simulink model "connecttoUDP_Ask_For_Ball"  (R2025a)
settings: Solver=ode4  StartTime=0.0  StopTime=inf  FixedStep=1/500  RelTol=1e-3  EnableMultiTasking=on
InitFcn:
  | home = [0.45; 0; 0.49];
  | pick = [0.3; 0; 0.3];
  | place = [-0.25; -0.25; 0.01];
  | waypoints = ...
  | [pick, pick,place ,place ,home]' ;
undefined symbols (not defined in the file): HIL, qc_get_step_size
libraries: quarc_library x18, simulink x3
(part 1 of 2)
settings Model: SimulationMode=external  ExtModeTrigDuration=10000  Creator=fvranes  LastModifiedBy=emano
settings SolverCC: AlgebraicLoopSolver=TrustRegion  PositivePriorityOrder=on
settings DataIOCC: SaveOutput=off  SignalLogging=off  DSMLogging=off  SaveTime=off  ReturnWorkspaceOutputs=off
settings OptimizationCC: ReuseModelBlockBuffer=off
settings DebuggingCC: UnconnectedInputMsg=warning  UnconnectedOutputMsg=warning  UnconnectedLineMsg=warning  ArithmeticOperatorsInVariantConditions=warning
settings ModelReferenceCC: EnableRefExpFcnMdlSchedulingChecks=on
settings SFSimCC: SimUseLocalCustomCode=off  CustomCodeUndefinedFunction=UseInterfaceOnly
settings RTWCC: SystemTargetFile=quarc_win64.tlc  TemplateMakefile=quarc_default_tmf  RTWUseLocalCustomCode=off  Toolchain=QUARC win64 | nmake (64-bit Windows)  BuildConfiguration=Faster Runs  GPUComputeCapability=3.5  Description=QUARC Win64 Target Using Toolchain
settings CodeAppCC: StateflowObjectComments=on
settings STFCustomTargetCC: SystemTargetFile=quarc_win64.tlc  TargetLangStandard=C99 (ISO)  MultiwordLength=2048.0  DynamicStringBufferSize=256.0  ConcurrentExecutionCompliant=on  UseToolchainInfoCompliant=on
settings GRTTargetCC: ExtMode=on  ExtModeMexFile=quarc_comm  ParMdlRefBuildCompliant=off  CompOptLevelCompliant=off  CombineOutputUpdateFcns=off  MatFileLogging=off  CPPClassGenCompliant=off  GRTInterface=on
settings ConfigComp: CovMetricSettings=dswe

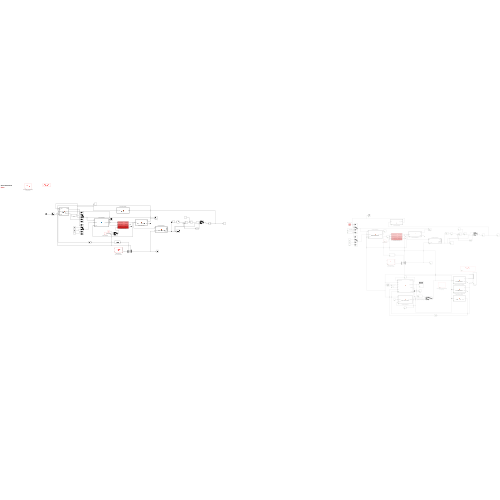
[thumbnail: Simulink's stored preview of the top-level diagram]
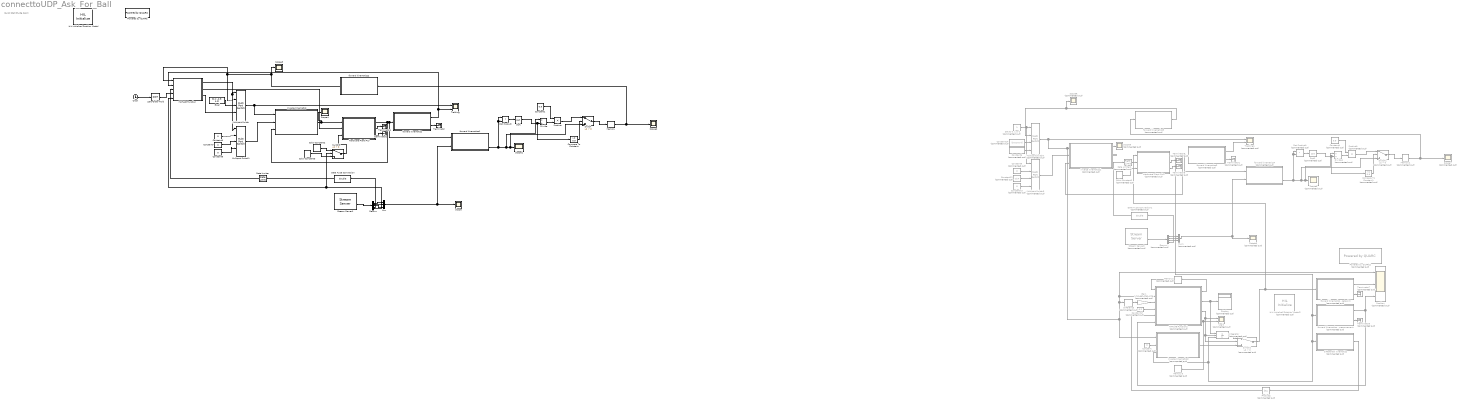
== system connecttoUDP_Ask_For_Ball ==
  note: Quick Start Guide
      | QArm
  Clock : Clock
  Color Constant1 : quarc_library/Sources/Signals/Color Constant  Commented=on  color=[0.71765 0.27451 1]
      settings: SourceProductName=QUARC Targets
  Color Constant2 : quarc_library/Sources/Signals/Color Constant  color=[0.23137 0.66667 0.19608]
      settings: SourceProductName=QUARC Targets
  Color Constant3 : quarc_library/Sources/Signals/Color Constant  color=[0.86667 0.32941 0]
      settings: SourceProductName=QUARC Targets
  Compare To Constant : simulink/Logic and Bit Operations/Compare To Constant  relop=>=  const=0.9  OutDataTypeStr=boolean
  Compare To Constant1 : simulink/Logic and Bit Operations/Compare To Constant  Commented=on  relop=>=  const=0.9  OutDataTypeStr=boolean
  Constant : Constant  Commented=on  Value=0
  Constant1 : Constant  Value=0.9
  Constant10 : Constant  Commented=on  Value=[0 0.5 0.4]
  Constant11 : Constant  Commented=on  Value=0.2
  Constant12 : Constant  Commented=on  Value=-pi/4
  Constant13 : Constant  Commented=on  Value=0
  Constant3 : Constant  Value=0
  Constant4 : Constant  Commented=on  Value=0.9
  Constant6 : Constant  Commented=on  Value=[0 -0.5*sin(pi/2) 0]
  Constant7 : Constant  Value=0
  Constant8 : Constant  Value=0
  Constant9 : Constant  Commented=on  Value=0
  Data Type Conversion : DataTypeConversion  OutMin=0  OutMax=11  OutDataTypeStr=double  SaturateOnIntegerOverflow=off  RndMeth=Floor
  Data Type Conversion1 : DataTypeConversion  Commented=on  OutMin=[0]  OutMax=1  OutDataTypeStr=double  SaturateOnIntegerOverflow=off  RndMeth=Floor
  Demux : Demux  Outputs=5
  Demux1 : Demux  Commented=on
  Difference : simulink/Discrete/Difference  Commented=on  ICPrevInput=0.0  OutMin=[]  OutMax=[]  OutDataType=fixdt(1, 16)  OutScaling=2^-10  DoSatur=off
  Display : Display  Commented=on
  Divide : Product  Inputs=*/
  Divide1 : Product  Commented=on  Inputs=*/
  Dot Product : DotProduct  OutDataTypeStr=Inherit: Inherit via internal rule
  Dot Product1 : DotProduct  Commented=on  OutDataTypeStr=Inherit: Inherit via internal rule
  Gain : Gain  Commented=on  Gain=1/qc_get_step_size
  Goal : Constant  Value=[0.2; -0.5; 0.2]
  HIL Initialize (Position Mode) : quarc_library/Data Acquisition/Generic/Configuration/HIL Initialize  object_name=HIL-1  board_type=qarm_usb  board_number=0  board_options=j0_mode=0;j1_mode=0;j2_mode=0;j3_mode=0;gripper_mode=0;j0_profile_config=0;j0_profile_velocity=1.5708;j0_profile_acceleration=1.0472;j1_profile_config=0;j1_profile_velocity=1.5708;j1_profile_acceleration=1.0472;j2_profile_config=0;j2_profile_velocity=1.5708;j2_profile_acceleration=1.0472;j3_profile_config=0;j3_profile_velocity=1.5708;j3_profile_acceleration=1.0472;  exclusive=off  active=on  hardware_clocks=[0]  clock_modes=[]  initial_clock_frequencies=[]  set_clock_params_at_start=off  set_clock_params_at_switch_in=off  set_clock_frequencies_at_start=off  set_clock_frequencies_at_switch_in=off  analog_input_channels=[5:9]  analog_input_configurations=[]  analog_input_maximums=[]  analog_input_minimums=[]  set_analog_input_params_at_start=off  set_analog_input_params_at_switch_in=off  analog_output_channels=[]  analog_output_maximums=inf  analog_output_minimums=-inf  initial_analog_outputs=[0]  final_analog_outputs=[0]  watchdog_analog_outputs=[]  set_analog_output_params_at_start=off  set_analog_output_params_at_switch_in=off  set_analog_outputs_at_start=off  set_analog_outputs_at_switch_in=off  set_analog_outputs_at_terminate=off  set_analog_outputs_at_switch_out=off  set_analog_outputs_on_watchdog=off  digital_input_channels=[]  digital_output_channels=[]  digital_output_configuration=[]  initial_digital_outputs=[0]  final_digital_outputs=[0]  watchdog_digital_outputs=[0]  set_digital_output_params_at_start=off  set_digital_output_params_at_switch_in=off  set_digital_outputs_at_start=off  set_digital_outputs_at_switch_in=off  set_digital_outputs_at_terminate=off  set_digital_outputs_at_switch_out=off  set_digital_outputs_on_watchdog=off  encoder_channels=[]  quadrature=[]  encoder_filter_frequency=[]  initial_encoder_counts=[]  set_encoder_params_at_start=off  set_encoder_params_at_switch_in=off  set_encoder_counts_at_start=off  set_encoder_counts_at_switch_in=off  pwm_channels=[]  pwm_modes=[]  pwm_frequency=[]  pwm_configuration=[]  pwm_alignment=[]  pwm_polarity=[]  pwm_leading_deadband=[]  pwm_trailing_deadband=[]  initial_pwm_outputs=[]  final_pwm_outputs=[]  watchdog_pwm_outputs=[]  set_pwm_params_at_start=off  set_pwm_params_at_switch_in=off  set_pwm_outputs_at_start=off  set_pwm_outputs_at_switch_in=off  set_pwm_outputs_at_terminate=off  set_pwm_outputs_at_switch_out=off  set_pwm_outputs_on_watchdog=off  other_output_channels=[1000:1004 11000:11003 11005:11007]  initial_other_outputs=[zeros(1,9), ones(1,3)]  final_other_outputs=[zeros(1,9), ones(1,3)]  watchdog_other_outputs=zeros(1,12)  set_other_outputs_at_start=off  set_other_outputs_at_switch_in=off  set_other_outputs_at_terminate=on  set_other_outputs_at_switch_out=off  set_other_outputs_on_watchdog=off
  HIL Initialize (Position Mode)2 : quarc_library/Data Acquisition/Generic/Configuration/HIL Initialize  Priority=1  Commented=on  object_name=HIL-2  board_type=qarm_usb  board_number=0  board_options=j0_mode=0;j1_mode=0;j2_mode=0;j3_mode=0;gripper_mode=0;j0_profile_config=0;j0_profile_velocity=0;j0_profile_acceleration=0;j1_profile_config=0;j1_profile_velocity=0;j1_profile_acceleration=0;j2_profile_config=0;j2_profile_velocity=0;j2_profile_acceleration=0;j3_profile_config=0;j3_profile_velocity=0;j3_profile_acceleration=0;  exclusive=off  active=on  hardware_clocks=[0]  clock_modes=[]  initial_clock_frequencies=[]  set_clock_params_at_start=off  set_clock_params_at_switch_in=off  set_clock_frequencies_at_start=off  set_clock_frequencies_at_switch_in=off  analog_input_channels=[5:9]  analog_input_configurations=[]  analog_input_maximums=[]  analog_input_minimums=[]  set_analog_input_params_at_start=off  set_analog_input_params_at_switch_in=off  analog_output_channels=[]  analog_output_maximums=inf  analog_output_minimums=-inf  initial_analog_outputs=[0]  final_analog_outputs=[0]  watchdog_analog_outputs=[]  set_analog_output_params_at_start=off  set_analog_output_params_at_switch_in=off  set_analog_outputs_at_start=off  set_analog_outputs_at_switch_in=off  set_analog_outputs_at_terminate=off  set_analog_outputs_at_switch_out=off  set_analog_outputs_on_watchdog=off  digital_input_channels=[]  digital_output_channels=[]  digital_output_configuration=[]  initial_digital_outputs=[0]  final_digital_outputs=[0]  watchdog_digital_outputs=[0]  set_digital_output_params_at_start=off  set_digital_output_params_at_switch_in=off  set_digital_outputs_at_start=off  set_digital_outputs_at_switch_in=off  set_digital_outputs_at_terminate=off  set_digital_outputs_at_switch_out=off  set_digital_outputs_on_watchdog=off  encoder_channels=[]  quadrature=[]  encoder_filter_frequency=[]  initial_encoder_counts=[]  set_encoder_params_at_start=off  set_encoder_params_at_switch_in=off  set_encoder_counts_at_start=off  set_encoder_counts_at_switch_in=off  pwm_channels=[]  pwm_modes=[]  pwm_frequency=[]  pwm_configuration=[]  pwm_alignment=[]  pwm_polarity=[]  pwm_leading_deadband=[]  pwm_trailing_deadband=[]  initial_pwm_outputs=[]  final_pwm_outputs=[]  watchdog_pwm_outputs=[]  set_pwm_params_at_start=off  set_pwm_params_at_switch_in=off  set_pwm_outputs_at_start=off  set_pwm_outputs_at_switch_in=off  set_pwm_outputs_at_terminate=off  set_pwm_outputs_at_switch_out=off  set_pwm_outputs_on_watchdog=off  other_output_channels=[1000:1004 11000:11003 11005:11007]  initial_other_outputs=[zeros(1,9), ones(1,3)]  final_other_outputs=[zeros(1,9), ones(1,3)]  watchdog_other_outputs=zeros(1,12)  set_other_outputs_at_start=off  set_other_outputs_at_switch_in=off  set_other_outputs_at_terminate=off  set_other_outputs_at_switch_out=off  set_other_outputs_on_watchdog=off
  Hardware Plant P(s) : Subsystem
  Hardware Plant P(s)1 : Subsystem  Commented=on
  Integrator : Integrator  Commented=on  ExternalReset=rising  InitialConditionSource=external  LimitOutput=on  UpperSaturationLimit=[170 85 85 180]*pi/180  LowerSaturationLimit=[-170 -85 -95 -180]*pi/180
  Logic : Scope  Commented=on  NumInputPorts=2
      settings: ActiveDisplayYMinimum=-0.125  ActiveDisplayYMaximum=1.125  DataLoggingVariableName=ScopeData8
  MATLAB Function : MATLAB Function  TreatAsAtomicUnit=on
  MATLAB Function2 : MATLAB Function  Commented=on  TreatAsAtomicUnit=on
  Memory : Memory  InitialCondition=[0 ,0.5 ,0.5]
  Memory1 : Memory  Commented=on  InitialCondition=[0 ,0.5 ,0.5]
  Memory2 : Memory  Commented=on  InitialCondition=1
  Memory3 : Memory  Commented=on  InitialCondition=1
  Multiport Switch : MultiPortSwitch  Inputs=4  SaturateOnIntegerOverflow=off  InputSameDT=off
  Multiport Switch1 : MultiPortSwitch  Inputs=4  SaturateOnIntegerOverflow=off  InputSameDT=off
  Multiport Switch2 : MultiPortSwitch  Commented=on  SaturateOnIntegerOverflow=off  InputSameDT=off
  Multiport Switch3 : MultiPortSwitch  Commented=on  SaturateOnIntegerOverflow=off  InputSameDT=off
  Mux : Mux  Inputs=3
  Mux1 : Mux  Commented=on  Inputs=3
  Position : Scope  Commented=on  NumInputPorts=3
      settings: TimeSpan=90  ActiveDisplayYMinimum=-0.58261  ActiveDisplayYMaximum=0.73336  DataLoggingVariableName=ScopeData9
  Powered by QUARC : quarc_library/Logos/Powered by QUARC
  Powered by QUARC2 : quarc_library/Logos/Powered by QUARC  Commented=on
  Product : Product
  Product1 : Product  Commented=on
  Product2 : Product  Commented=on  Inputs=/  Multiplication=Matrix(*)
  Rate Limiter : RateLimiter  SampleTimeMode=inherited
  Rate Limiter1 : RateLimiter  Commented=on  SampleTimeMode=inherited
  Scope{,1..4} (5 alike) : Scope
      Scope settings: ActiveDisplayYMinimum=-0.053062727209180587  ActiveDisplayYMaximum=0.31034032395109534  DataLoggingVariableName=ScopeData2
      Scope1 settings: ActiveDisplayYMinimum=-0.12497992207214531  ActiveDisplayYMaximum=2.6391843046872321
      Scope2 settings: ActiveDisplayYMinimum=-0.15530750088098816  ActiveDisplayYMaximum=0.15932707853928335  DataLoggingVariableName=ScopeData3
      Scope3 settings: ActiveDisplayYMinimum=-0.2741132612100553  ActiveDisplayYMaximum=0.52763613707129164  DataLoggingVariableName=ScopeData6
      Scope4 settings: ActiveDisplayYMinimum=-1.68864453030744  ActiveDisplayYMaximum=2.6969512581912602  DataLoggingVariableName=ScopeData7
  Scope{5..9} (5 alike) : Scope  Commented=on
      Scope5 settings: ActiveDisplayYMinimum=-0.053062727209180587  ActiveDisplayYMaximum=0.31034032395109534  DataLoggingVariableName=ScopeData10
      Scope6 settings: ActiveDisplayYMinimum=-0.12497992207214531  ActiveDisplayYMaximum=2.6391843046872321  DataLoggingVariableName=ScopeData11
      Scope7 settings: ActiveDisplayYMinimum=-0.15530750088098816  ActiveDisplayYMaximum=0.15932707853928335  DataLoggingVariableName=ScopeData12
      Scope8 settings: ActiveDisplayYMinimum=-0.2741132612100553  ActiveDisplayYMaximum=0.52763613707129164  DataLoggingVariableName=ScopeData13
      Scope9 settings: ActiveDisplayYMinimum=-1.68864453030744  ActiveDisplayYMaximum=2.6969512581912602  DataLoggingVariableName=ScopeData14
  "Set to 0, 1 or 1" : Constant  Commented=on
  Sqrt : Sqrt
  Sqrt1 : Sqrt  Commented=on
  Stream Server1 : quarc_library/Communications/Basic/Stream Server  uri_source=Specify via dialog (do not evaluate)  uri=udp://localhost:5005  send_buffer_size=1460  receive_buffer_size=1460  byte_order=little endian (Intel - LSB first)  optimization=Minimum latency  send_options=Send all data  receive_options=Receive all data  default_value=[0,0,0,0,0]  sample_time=qc_get_step_size  active=off  implementation=Use blocking I/O in a separate thread  send_fifo_size=1000  receive_fifo_size=1000  send_priority=0  receive_priority=0  send_dimensions=off  receive_dimensions=off  max_dimensions=-1  data_type=single  type_expr=BusObject
      settings: AttributesFormatString="\"udp://localhost:5005\""
  Stream Server2 : quarc_library/Communications/Basic/Stream Server  Commented=on  uri_source=Specify via dialog (do not evaluate)  uri=udp://localhost:5005  send_buffer_size=1460  receive_buffer_size=1460  byte_order=little endian (Intel - LSB first)  optimization=Minimum latency  send_options=Send all data  receive_options=Receive all data  default_value=[0,0,0,0]  sample_time=qc_get_step_size  active=off  implementation=Use blocking I/O in a separate thread  send_fifo_size=1000  receive_fifo_size=1000  send_priority=0  receive_priority=0  send_dimensions=off  receive_dimensions=off  max_dimensions=-1  data_type=single  type_expr=BusObject
      settings: AttributesFormatString="\"udp://localhost:5005\""
  Switch : Switch  Criteria=u2 > Threshold  SaturateOnIntegerOverflow=off  InputSameDT=off
  Switch1 : Switch  Commented=on  Criteria=u2 > Threshold  SaturateOnIntegerOverflow=off  InputSameDT=off
  Switch2 : Switch  Commented=on  Criteria=u2 > Threshold  SaturateOnIntegerOverflow=off  InputSameDT=off
  Switch3 : Switch  Criteria=u2 > Threshold  SaturateOnIntegerOverflow=off  InputSameDT=off
  Terminator : Terminator
  Terminator{1,3,5..7} (5 alike) : Terminator  Commented=on
  Terminator2 : Terminator
  Terminator4 : Terminator
  Tracking : Scope  NumInputPorts=2
      settings: ActiveDisplayYMinimum=0.07139  ActiveDisplayYMaximum=0.54944
  Tracking1 : Scope  Commented=on  NumInputPorts=2
      settings: ActiveDisplayYMinimum=0.07139  ActiveDisplayYMaximum=0.54944  DataLoggingVariableName=ScopeData15
  Zero-Order Hold : ZeroOrderHold  SampleTime=-1
  differential kinematics : MATLAB Function  Commented=on  TreatAsAtomicUnit=on
  forward kinematics : MATLAB Function  TreatAsAtomicUnit=on
  forward kinematics - measurement : MATLAB Function  Commented=on  TreatAsAtomicUnit=on
  forward kinematics - setpoint : MATLAB Function  Commented=on  TreatAsAtomicUnit=on
  forward kinematics1 : MATLAB Function  TreatAsAtomicUnit=on
  forward kinematics2 : MATLAB Function  TreatAsAtomicUnit=on
  forward kinematics3 : MATLAB Function  Commented=on  TreatAsAtomicUnit=on
  forward kinematics4 : MATLAB Function  Commented=on  TreatAsAtomicUnit=on
  forward kinematics5 : MATLAB Function  Commented=on  TreatAsAtomicUnit=on
  inverse kinematics : MATLAB Function  TreatAsAtomicUnit=on
  inverse kinematics1 : MATLAB Function  Commented=on  TreatAsAtomicUnit=on
  inverse kinematics2 : MATLAB Function  Commented=on  TreatAsAtomicUnit=on
  wires:
  forward kinematics/2(R04) -> Terminator/1
  inverse kinematics/1(phi_optimal) -> Scope4/1, Hardware Plant P(s)/1(Phi Cmd (rad) [4])
  Demux/4 -> Data Type Conversion/1
  Constant7/1 -> Multiport Switch1/3
  Multiport Switch1/1 -> inverse kinematics/2(gamma)
  MATLAB Function/1(number) -> Multiport Switch1/1, Multiport Switch/1
  Multiport Switch/1 -> inverse kinematics/1(p), Tracking/1
  MATLAB Function/3(search_pos) -> Multiport Switch/4
  forward kinematics/1(p4) -> Tracking/2, MATLAB Function/2(p4)
  Hardware Plant P(s)/3(PWM (%) [4]) -> Terminator2/1
  Constant8/1 -> Multiport Switch1/4
  Hardware Plant P(s)/2(Gripper (%)) -> Terminator4/1
  Constant3/1 -> Multiport Switch1/2
  forward kinematics1/6(p_obj_0) -> Dot Product/1, Dot Product/2, Switch/3, Divide/1, Scope1/1
  Hardware Plant P(s)/1(Phi (rad) [4]) -> forward kinematics1/1(phi), forward kinematics/1(phi), inverse kinematics/3(phi_prev)
  Stream Server1/4 -> Demux/1
  Dot Product/1 -> Sqrt/1
  Sqrt/1 -> Compare To Constant/1, Divide/2
  Divide/1 -> Product/2
  Constant1/1 -> Product/1
  Product/1 -> Switch/1
  Compare To Constant/1 -> Switch/2
  Switch/1 -> Memory/1
  Memory/1 -> forward kinematics2/1(xyz), Scope2/1
  forward kinematics2/1(xyz_mean) -> Scope3/1, Multiport Switch/2, MATLAB Function/1(xyz_mean)
  Mux/1 -> forward kinematics1/2(p_obj_cam), Scope/1
  Demux/1 -> Mux/1
  Demux/2 -> Mux/2
  Demux/3 -> Mux/3
  Data Type Conversion/1 -> Rate Limiter/1
  Switch2/1 -> Hardware Plant P(s)1/1(Phi Cmd (rad) [4]), forward kinematics - setpoint/1(phi)
  forward kinematics - measurement/2(R04) -> Terminator3/1
  MATLAB Function2/1(next_state) -> Memory2/1
  Difference/1 -> Gain/1
  Gain/1 -> MATLAB Function2/3(vT)
  forward kinematics - setpoint/1(p4) -> Position/2  "commanded"
  MATLAB Function2/3(avoiding) -> Switch2/2, Integrator/2, Logic/1
  Demux1/3 -> Mux1/3
  Data Type Conversion1/1 -> Rate Limiter1/1
  Demux1/4 -> Data Type Conversion1/1
  Integrator/1 -> Switch2/1
  differential kinematics/1(J) -> Product2/1
  Memory2/1 -> MATLAB Function2/1(current_state)
  Mux1/1 -> Scope5/1, forward kinematics4/2(p_obj_cam)
  inverse kinematics2/1(phi_optimal) -> Switch2/3  "physical joint angles (phi)"
  forward kinematics - setpoint/2(R04) -> Terminator7/1
  Product2/1 -> MATLAB Function2/5(invJ)
  Constant/1 -> inverse kinematics2/2(gamma)
  MATLAB Function2/4(pause) -> Memory3/1, Logic/2
  forward kinematics - measurement/1(p4) -> Position/3, MATLAB Function2/6(pM)  "measured"
  Demux1/1 -> Mux1/1
  Constant11/1 -> MATLAB Function2/4(R)
  Divide1/1 -> Product1/2
  forward kinematics4/6(p_obj_0) -> Dot Product1/1, Dot Product1/2, Switch1/3, Divide1/1, Scope6/1
  Hardware Plant P(s)1/3(PWM (%) [4]) -> Terminator5/1
  Hardware Plant P(s)1/1(Phi (rad) [4]) -> forward kinematics4/1(phi), forward kinematics3/1(phi), inverse kinematics1/3(phi_prev), differential kinematics/1(phi), inverse kinematics2/3(phi_prev), Integrator/3, forward kinematics - measurement/1(phi)
  Constant12/1 -> Multiport Switch3/3
  Constant4/1 -> Product1/1
  forward kinematics3/1(p4) -> Tracking1/2
  Multiport Switch3/1 -> inverse kinematics1/2(gamma)
  Color Constant1/1 -> Hardware Plant P(s)1/3(Base RGB Led (%))
  Switch1/1 -> Memory1/1
  Dot Product1/1 -> Sqrt1/1
  inverse kinematics1/1(phi_optimal) -> Scope9/1
  Product1/1 -> Switch1/1
  forward kinematics3/2(R04) -> Terminator1/1
  Constant13/1 -> Multiport Switch3/4
  Constant10/1 -> Multiport Switch2/3
  Compare To Constant1/1 -> Switch1/2
  "Set to 0, 1 or 1"/1 -> Multiport Switch3/1, Multiport Switch2/1
  Hardware Plant P(s)1/2(Gripper (%)) -> Terminator6/1
  Rate Limiter1/1 -> Hardware Plant P(s)1/2(Gripper Cmd (0,1))
  Sqrt1/1 -> Compare To Constant1/1, Divide1/2
  MATLAB Function2/2(phi_speed) -> Integrator/1, Display/1
  Constant9/1 -> Multiport Switch3/2
  forward kinematics5/1(xyz_mean) -> Scope8/1, Multiport Switch2/2
  Constant6/1 -> Multiport Switch2/4
  Multiport Switch2/1 -> inverse kinematics2/1(p), Position/1, MATLAB Function2/2(pT), Difference/1, inverse kinematics1/1(p), Tracking1/1  "desired"
  Memory1/1 -> forward kinematics5/1(xyz), Scope7/1
  Demux1/2 -> Mux1/2
  Stream Server2/4 -> Demux1/1
  Rate Limiter/1 -> MATLAB Function/3(python_cmd)
  MATLAB Function/2(gripper_cmd) -> Hardware Plant P(s)/2(Gripper Cmd (0,1))
  Goal/1 -> Multiport Switch/3
  Clock/1 -> Zero-Order Hold/1
  Zero-Order Hold/1 -> MATLAB Function/4(t)
  Demux/5 -> Switch3/2, MATLAB Function/5(is_visible)
  Switch3/1 -> Hardware Plant P(s)/3(Base RGB Led (%))
  Color Constant2/1 -> Switch3/1
  Color Constant3/1 -> Switch3/3

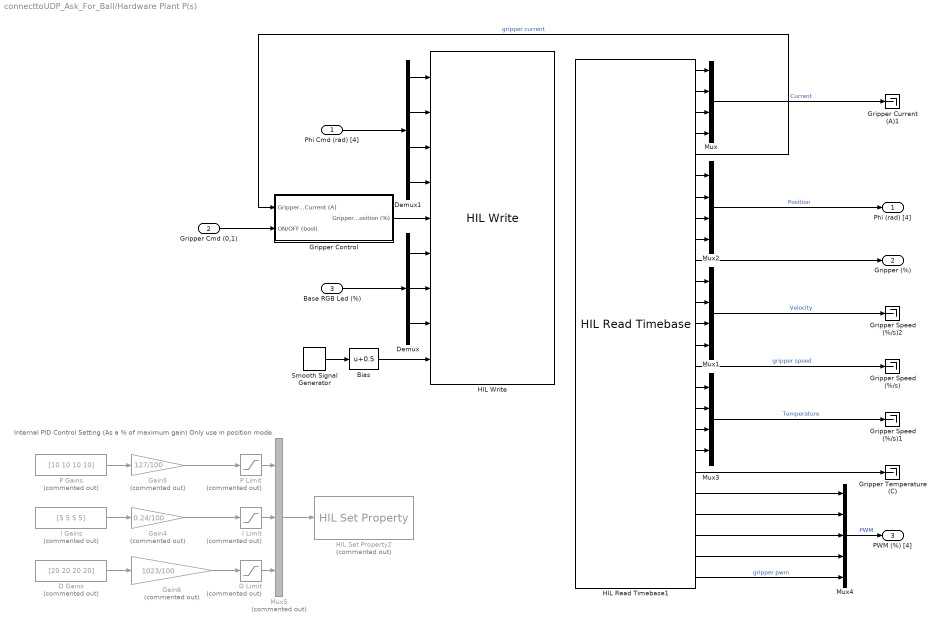
== system connecttoUDP_Ask_For_Ball/Hardware Plant P(s) ==
  note: Internal PID Control Setting (As a % of maximum gain)
      | Only use in position mode
  Phi Cmd (rad) [4] : Inport
  Gripper Cmd (0,1) : Inport  Port=2
  Base RGB Led (%) : Inport  Port=3
  Bias : Bias  Bias=0.5  SaturateOnIntegerOverflow=off
  D Gains : Constant  Commented=on  Value=[20 20 20 20]
  D Limit : Saturate  Commented=on  UpperLimit=[1023 1023 1023 1023]  LowerLimit=[0 0 0 0]
  Demux : Demux  Outputs=3
  Demux1 : Demux
  Gain4 : Gain  Commented=on  Gain=0.24/100
  Gain5 : Gain  Commented=on  Gain=127/100
  Gain6 : Gain  Commented=on  Gain=1023/100
  Gripper Control : Subsystem
  Gripper Current (A)1 : Terminator
  Gripper Speed (%/s) : Terminator
  Gripper Speed (%/s)1 : Terminator
  Gripper Speed (%/s)2 : Terminator
  Gripper Temperature (C) : Terminator
  HIL Read Timebase1 : quarc_library/Data Acquisition/Generic/Timebases/HIL Read Timebase  object_name=HIL-1  clock=0  analog_channels=[5:9]  encoder_channels=[]  digital_channels=[]  other_channels=[1000:1004 3000:3004 10000:10004 11000:11004]  active=on  vector_output=off  data_type_mode=Inherit via back propagation  encoder_data_type=double  digital_data_type=boolean  overflow_mode=Error on overflow  samples_in_buffer=max(ceil(1/qc_get_step_size), 1)
  HIL Set Property2 : quarc_library/Data Acquisition/Generic/Configuration/HIL Set Property  Commented=on  object_name=HIL-1  property_type=2  property_codes=[128:131 133:136 138:141]  property_source=2  property_value_num=0  set_at_start=on  sample_time=-1  active=off
      settings: AttributesFormatString=(%<object_name>)  SourceProductName=QUARC Targets
  HIL Write : quarc_library/Data Acquisition/Generic/Immediate I//O/HIL Write  object_name=HIL-1  analog_channels=[]  pwm_channels=[]  digital_channels=[]  other_channels=[1000:1004 11005:11008]  sample_time=-1  active=on  vector_input=off
  I Gains : Constant  Commented=on  Value=[5 5 5 5]
  I Limit : Saturate  Commented=on  UpperLimit=[0.24 0.24 0.24 0.24]  LowerLimit=[0 0 0 0]
  Mux{,1..3} (4 alike) : Mux
  Mux4 : Mux  Inputs=5
  Mux5 : Mux  Commented=on  Inputs=3
  P Gains : Constant  Commented=on  Value=[10 10 10 10]
  P Limit : Saturate  Commented=on  UpperLimit=[127 127 127 127]  LowerLimit=[0 0 0 0]
  Smooth Signal Generator : quarc_library/Sources/Signals/Smooth Signal Generator  signal_type=Sine  source=Internal (dialog parameters)  amplitude=0.5  frequency=60/72  initial_phase=0  sample_time=qc_get_step_size  output_cos=off
      settings: SourceProductName=QUARC Targets
  Phi (rad) [4] : Outport  VectorParamsAs1DForOutWhenUnconnected=off
  Gripper (%) : Outport  Port=2  VectorParamsAs1DForOutWhenUnconnected=off
  PWM (%) [4] : Outport  Port=3  VectorParamsAs1DForOutWhenUnconnected=off
  wires:
  HIL Read Timebase1/10 -> Gripper (%)/1
  Mux4/1 -> PWM (%) [4]/1  "PWM"
  HIL Read Timebase1/25 -> Mux4/5  "gripper pwm"
  HIL Read Timebase1/24 -> Mux4/4
  HIL Read Timebase1/23 -> Mux4/3
  HIL Read Timebase1/22 -> Mux4/2
  HIL Read Timebase1/21 -> Mux4/1
  Mux2/1 -> Phi (rad) [4]/1  "Position"
  Phi Cmd (rad) [4]/1 -> Demux1/1
  Demux1/4 -> HIL Write/4
  Demux1/3 -> HIL Write/3
  Demux1/2 -> HIL Write/2
  Demux1/1 -> HIL Write/1
  Base RGB Led (%)/1 -> Demux/1
  Mux3/1 -> Gripper Speed (%/s)1/1  "Temperature"
  Mux1/1 -> Gripper Speed (%/s)2/1  "Velocity"
  Mux/1 -> Gripper Current (A)1/1  "Current"
  HIL Read Timebase1/20 -> Gripper Temperature (C)/1
  HIL Read Timebase1/1 -> Mux/1
  HIL Read Timebase1/2 -> Mux/2
  HIL Read Timebase1/13 -> Mux1/3
  Demux/2 -> HIL Write/7
  HIL Read Timebase1/19 -> Mux3/4
  Demux/1 -> HIL Write/6
  HIL Read Timebase1/11 -> Mux1/1
  HIL Read Timebase1/16 -> Mux3/1
  HIL Read Timebase1/17 -> Mux3/2
  HIL Read Timebase1/3 -> Mux/3
  Demux/3 -> HIL Write/8
  HIL Read Timebase1/15 -> Gripper Speed (%/s)/1  "gripper speed"
  HIL Read Timebase1/5 -> Gripper Control/1(Gripper Current (A))  "gripper current"
  HIL Read Timebase1/7 -> Mux2/2
  HIL Read Timebase1/4 -> Mux/4
  HIL Read Timebase1/12 -> Mux1/2
  HIL Read Timebase1/8 -> Mux2/3
  HIL Read Timebase1/18 -> Mux3/3
  HIL Read Timebase1/6 -> Mux2/1
  HIL Read Timebase1/9 -> Mux2/4
  HIL Read Timebase1/14 -> Mux1/4
  Gripper Control/1(Gripper Position (%)) -> HIL Write/5
  Gripper Cmd (0,1)/1 -> Gripper Control/2(ON/OFF (bool))
  Smooth Signal Generator/1 -> Bias/1
  Bias/1 -> HIL Write/9
  I Limit/1 -> Mux5/2
  Gain5/1 -> P Limit/1
  D Limit/1 -> Mux5/3
  Mux5/1 -> HIL Set Property2/1
  I Gains/1 -> Gain4/1
  P Gains/1 -> Gain5/1
  D Gains/1 -> Gain6/1
  P Limit/1 -> Mux5/1
  Gain6/1 -> D Limit/1
  Gain4/1 -> I Limit/1

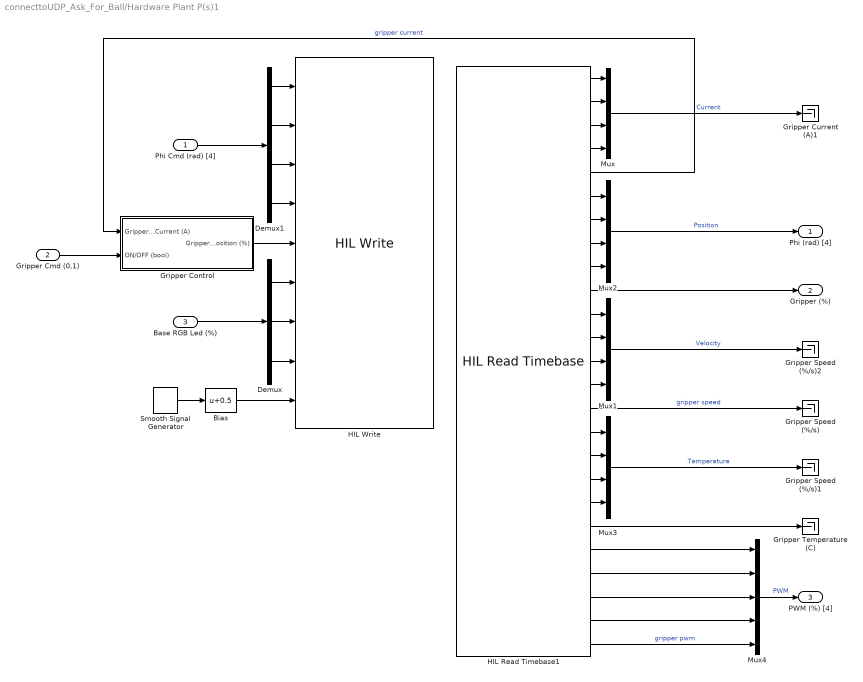
== system connecttoUDP_Ask_For_Ball/Hardware Plant P(s)1 ==
  Phi Cmd (rad) [4] : Inport
  Gripper Cmd (0,1) : Inport  Port=2
  Base RGB Led (%) : Inport  Port=3
  Bias : Bias  Bias=0.5  SaturateOnIntegerOverflow=off
  Demux : Demux  Outputs=3
  Demux1 : Demux
  Gripper Control : Subsystem
  Gripper Current (A)1 : Terminator
  Gripper Speed (%/s) : Terminator
  Gripper Speed (%/s)1 : Terminator
  Gripper Speed (%/s)2 : Terminator
  Gripper Temperature (C) : Terminator
  HIL Read Timebase1 : quarc_library/Data Acquisition/Generic/Timebases/HIL Read Timebase  object_name=unassigned  clock=0  analog_channels=[5:9]  encoder_channels=[]  digital_channels=[]  other_channels=[1000:1004 3000:3004 10000:10004 11000:11004]  active=on  vector_output=off  data_type_mode=Inherit via back propagation  encoder_data_type=double  digital_data_type=boolean  overflow_mode=Error on overflow  samples_in_buffer=max(ceil(1/qc_get_step_size), 1)
  HIL Write : quarc_library/Data Acquisition/Generic/Immediate I//O/HIL Write  object_name=unassigned  analog_channels=[]  pwm_channels=[]  digital_channels=[]  other_channels=[1000:1004 11005:11008]  sample_time=-1  active=on  vector_input=off
  Mux{,1..3} (4 alike) : Mux
  Mux4 : Mux  Inputs=5
  Smooth Signal Generator : quarc_library/Sources/Signals/Smooth Signal Generator  signal_type=Sine  source=Internal (dialog parameters)  amplitude=0.5  frequency=60/72  initial_phase=0  sample_time=qc_get_step_size  output_cos=off
      settings: SourceProductName=QUARC Targets
  Phi (rad) [4] : Outport  VectorParamsAs1DForOutWhenUnconnected=off
  Gripper (%) : Outport  Port=2  VectorParamsAs1DForOutWhenUnconnected=off
  PWM (%) [4] : Outport  Port=3  VectorParamsAs1DForOutWhenUnconnected=off
  wires:
  HIL Read Timebase1/10 -> Gripper (%)/1
  Mux4/1 -> PWM (%) [4]/1  "PWM"
  HIL Read Timebase1/25 -> Mux4/5  "gripper pwm"
  HIL Read Timebase1/24 -> Mux4/4
  HIL Read Timebase1/23 -> Mux4/3
  HIL Read Timebase1/22 -> Mux4/2
  HIL Read Timebase1/21 -> Mux4/1
  Mux2/1 -> Phi (rad) [4]/1  "Position"
  Phi Cmd (rad) [4]/1 -> Demux1/1
  Demux1/4 -> HIL Write/4
  Demux1/3 -> HIL Write/3
  Demux1/2 -> HIL Write/2
  Demux1/1 -> HIL Write/1
  Base RGB Led (%)/1 -> Demux/1
  Mux3/1 -> Gripper Speed (%/s)1/1  "Temperature"
  Mux1/1 -> Gripper Speed (%/s)2/1  "Velocity"
  Mux/1 -> Gripper Current (A)1/1  "Current"
  HIL Read Timebase1/20 -> Gripper Temperature (C)/1
  HIL Read Timebase1/1 -> Mux/1
  HIL Read Timebase1/2 -> Mux/2
  HIL Read Timebase1/13 -> Mux1/3
  Demux/2 -> HIL Write/7
  HIL Read Timebase1/19 -> Mux3/4
  Demux/1 -> HIL Write/6
  HIL Read Timebase1/11 -> Mux1/1
  HIL Read Timebase1/16 -> Mux3/1
  HIL Read Timebase1/17 -> Mux3/2
  HIL Read Timebase1/3 -> Mux/3
  Demux/3 -> HIL Write/8
  HIL Read Timebase1/15 -> Gripper Speed (%/s)/1  "gripper speed"
  HIL Read Timebase1/5 -> Gripper Control/1(Gripper Current (A))  "gripper current"
  HIL Read Timebase1/7 -> Mux2/2
  HIL Read Timebase1/4 -> Mux/4
  HIL Read Timebase1/12 -> Mux1/2
  HIL Read Timebase1/8 -> Mux2/3
  HIL Read Timebase1/18 -> Mux3/3
  HIL Read Timebase1/6 -> Mux2/1
  HIL Read Timebase1/9 -> Mux2/4
  HIL Read Timebase1/14 -> Mux1/4
  Gripper Control/1(Gripper Position (%)) -> HIL Write/5
  Gripper Cmd (0,1)/1 -> Gripper Control/2(ON/OFF (bool))
  Smooth Signal Generator/1 -> Bias/1
  Bias/1 -> HIL Write/9

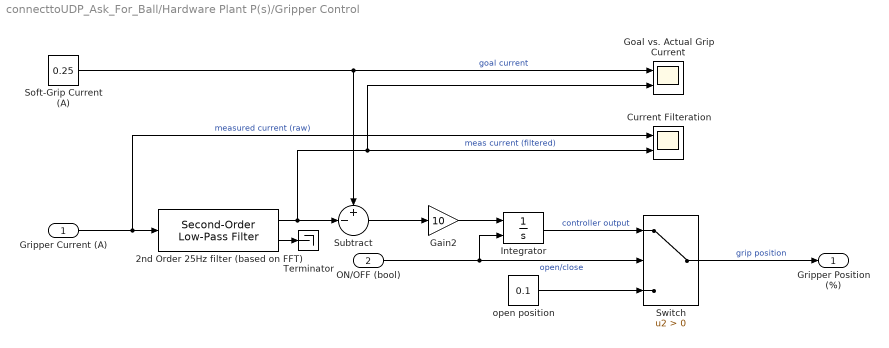
== system connecttoUDP_Ask_For_Ball/Hardware Plant P(s)/Gripper Control ==
  Gripper Current (A) : Inport
  ON/OFF (bool) : Inport  Port=2
  2nd Order 25Hz filter (based on FFT) : quarc_library/Continuous/Second-Order Low-Pass Filter  params_source=Internal (dialog parameters)  input_width=25*2*pi  input_zeta=1  input_init=0
  Current Filteration : Scope  NumInputPorts=2
      settings: ActiveDisplayYMinimum=-0.01447  ActiveDisplayYMaximum=0.62651  DataLoggingVariableName=ScopeData5
  Gain2 : Gain  Gain=10
  Goal vs. Actual Grip Current : Scope  NumInputPorts=2
      settings: ActiveDisplayYMinimum=0.00229  ActiveDisplayYMaximum=0.27702  DataLoggingVariableName=ScopeData4
  Integrator : Integrator  ExternalReset=either  InitialCondition=0.1  LimitOutput=on  UpperSaturationLimit=0.9  LowerSaturationLimit=0.1
  Soft-Grip Current (A) : Constant  Value=0.25
  Subtract : Sum  Inputs=+-|
  Switch : Switch  Criteria=u2 > Threshold  SaturateOnIntegerOverflow=off  InputSameDT=off
  Terminator : Terminator
  open position : Constant  Value=0.1
  Gripper Position (%) : Outport  VectorParamsAs1DForOutWhenUnconnected=off
  wires:
  Gripper Current (A)/1 -> 2nd Order 25Hz filter (based on FFT)/1, Current Filteration/1  "measured current (raw)"
  ON/OFF (bool)/1 -> Switch/2, Integrator/2  "open/close"
  open position/1 -> Switch/3
  Switch/1 -> Gripper Position (%)/1  "grip position"
  Soft-Grip Current (A)/1 -> Subtract/1, Goal vs. Actual Grip Current/1  "goal current"
  2nd Order 25Hz filter (based on FFT)/1 -> Subtract/2, Current Filteration/2, Goal vs. Actual Grip Current/2  "meas current (filtered)"
  Subtract/1 -> Gain2/1
  Integrator/1 -> Switch/1  "controller output"
  Gain2/1 -> Integrator/1
  2nd Order 25Hz filter (based on FFT)/2 -> Terminator/1

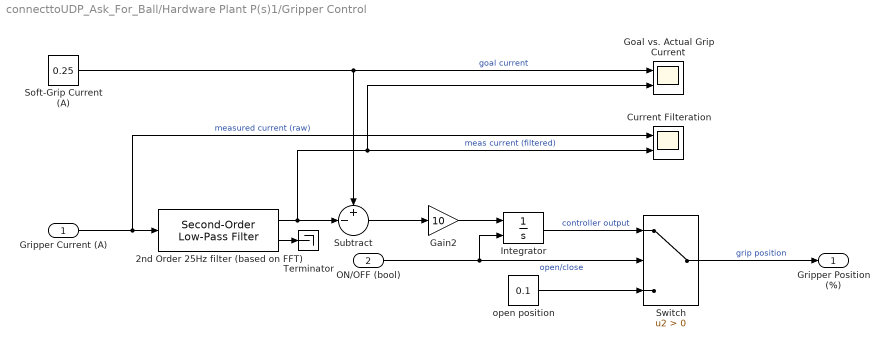
== system connecttoUDP_Ask_For_Ball/Hardware Plant P(s)1/Gripper Control ==
  Gripper Current (A) : Inport
  ON/OFF (bool) : Inport  Port=2
  2nd Order 25Hz filter (based on FFT) : quarc_library/Continuous/Second-Order Low-Pass Filter  params_source=Internal (dialog parameters)  input_width=25*2*pi  input_zeta=1  input_init=0
  Current Filteration : Scope  NumInputPorts=2
      settings: ActiveDisplayYMinimum=-0.01447  ActiveDisplayYMaximum=0.62651  DataLoggingVariableName=ScopeData5
  Gain2 : Gain  Gain=10
  Goal vs. Actual Grip Current : Scope  NumInputPorts=2
      settings: ActiveDisplayYMinimum=0.00229  ActiveDisplayYMaximum=0.27702  DataLoggingVariableName=ScopeData4
  Integrator : Integrator  ExternalReset=either  InitialCondition=0.1  LimitOutput=on  UpperSaturationLimit=0.9  LowerSaturationLimit=0.1
  Soft-Grip Current (A) : Constant  Value=0.25
  Subtract : Sum  Inputs=+-|
  Switch : Switch  Criteria=u2 > Threshold  SaturateOnIntegerOverflow=off  InputSameDT=off
  Terminator : Terminator
  open position : Constant  Value=0.1
  Gripper Position (%) : Outport  VectorParamsAs1DForOutWhenUnconnected=off
  wires:
  Gripper Current (A)/1 -> 2nd Order 25Hz filter (based on FFT)/1, Current Filteration/1  "measured current (raw)"
  ON/OFF (bool)/1 -> Switch/2, Integrator/2  "open/close"
  open position/1 -> Switch/3
  Switch/1 -> Gripper Position (%)/1  "grip position"
  Soft-Grip Current (A)/1 -> Subtract/1, Goal vs. Actual Grip Current/1  "goal current"
  2nd Order 25Hz filter (based on FFT)/1 -> Subtract/2, Current Filteration/2, Goal vs. Actual Grip Current/2  "meas current (filtered)"
  Subtract/1 -> Gain2/1
  Integrator/1 -> Switch/1  "controller output"
  Gain2/1 -> Integrator/1
  2nd Order 25Hz filter (based on FFT)/2 -> Terminator/1

== matlab function connecttoUDP_Ask_For_Ball/MATLAB Function2 ==
  settings: updateMethod=DISCRETE
  data: next_state output; phi_speed output; avoiding output size=1; current_state input; pT input; vT input; R input; invJ input; pM input; pause output
function [next_state, phi_speed, avoiding, pause] = stateMachine(current_state, pT, vT, R, invJ, pM)

persistent rate output
if isempty(rate)
    rate = 0;
    output = [0;0;0];
end
pause = 0;
insideCircle = norm(pT(1:2),2) <= R;

switch current_state
    
    % Outside Avoidance Zone
    case 1 
        % State Transition
        if insideCircle
            next_state = 2;
        else
            next_state = 1;
        end
        
        % State Action
        phi_speed = [0; 0; 0; 0] ; 
        avoiding =0 ;
    
	% Move to target
    case 2 
        % State Computation Logic
        allRoots = roots([vT(1)^2+vT(2)^2, 2*(vT(1)*pT(1)+vT(2)*pT(2)), pT(1)^2 + pT(2)^2 - R^2]);
        solutions = real(allRoots);
        idx = 1;
        if solutions(2) >= solutions(1)
            idx = 2;
        end
        maxTime = max(solutions(idx), 0.002);
        output = [pT(1:2,1) + vT(1:2,1)*maxTime; pT(3)];
        maxAngle = atan2(output(2), output(1)) - atan2(pT(2), pT(1));          
        rate = maxAngle/maxTime;

        % State Transition
        next_state =3 ;
        
        % State Action
        phi_speed = [rate; 0; 0; 0];
        avoiding =1 ;
    
	% Wait at target
    case 3 
        % State Computation Logic (if target is close to output, wait for
        % arm to get close first befor proceeding)
%         if norm(pT - output, 2) < 0.001
%             pause = 1;
%         end
        
        % State Transition
        if norm(pM - output, 2) < 0.01
            next_state = 4;
        else
            next_state = 3;            
        end
        
        % State Action
        phi_speed = [rate; 0; 0; 0] ;
        avoiding = 1;
	
	% Exit Strategy
    case 4 
        % State Transition
        if norm(pT(1:2), 2) > R
            next_state = 1;
        else
            next_state = 4;
        end
        
        % State Action
        phi_speed = [0; 0; 0; 0] ;
        avoiding = 1 ;
	
	% Default Case
    otherwise
        % State Transition
        next_state = current_state;    
        
        % State Action
        phi_speed = [0; 0; 0; 0];
        avoiding = 0;
        
end

== matlab function connecttoUDP_Ask_For_Ball/forward kinematics4 ==
  data: p3 output; R03 output; phi input; p4 output; R04 output; p_cam_0 output; p_obj_0 output; p_obj_cam input
function [p3, R03, p4, R04, p_cam_0,p_obj_0] = qarmForwardKinematics(phi,p_obj_cam)

%% QUANSER_ARM_FPK
% v 4.0 - 4th June 2020

% REFERENCE: 
% Chapter 3. Forward Kinematics
% Robot Dynamics and Control 
% Spong, Vidyasagar
% 1989

% INPUTS:
% phi     : Alternate joint angles vector 4 x 1

% OUTPUTS:
% p4      : End-effector frame {4} position vector expressed in base frame {0}
% R04     : rotation matrix from end-effector frame {4} to base frame {0}

%% Manipulator parameters:
L1 = 0.1400;
L2 = 0.3500;
L3 = 0.0500;
L4 = 0.2500;
L5 = 0.1500;

%% Alternate parameters
l1 = L1;
l2 = sqrt(L2^2 + L3^2);
l3 = L4 + L5;
beta = atan(L3/L2);

%% From phi space to theta space 
theta = phi;
theta(1) = phi(1);
theta(2) = phi(2) + beta - pi/2;
theta(3) = phi(3) - beta;
theta(4) = phi(4);

%% Transformation matrices for all frames:

% T{i-1}{i} = quanser_arm_DH(  a, alpha,  d,     theta );
        T01 = quanser_arm_DH(  0, -pi/2, l1,  theta(1) );
        T12 = quanser_arm_DH( l2,     0,  0,  theta(2) );
        T23 = quanser_arm_DH(  0, -pi/2,  0,  theta(3) );
        T34 = quanser_arm_DH(  0,     0, l3,  theta(4) );

        T02 = T01*T12;
        T03 = T02*T23;
        T04 = T03*T34;

%% Position of end-effector Transformation

% Extract the Position vector 
% p1   = T01(1:3,4);
% p2   = T02(1:3,4);
p3   = T03(1:3,4);
p4   = T04(1:3,4);

% Extract the Rotation matrix
% R01 = T01(1:3,1:3);
% R02 = T02(1:3,1:3);
R03 = T03(1:3,1:3);
R04 = T04(1:3,1:3);

d_tilde = 0.3; % distance entre P03 et la caméra (m)

% position de la caméra dans le frame de l'articulation 3
p_cam_3 = [0; 0; d_tilde]; 

% position de la caméra dans le frame global {0}
p_cam_0 = p3 + R03 * p_cam_3;

R_cam_3 = [ -1  0  0;
             0  1  0;
             0  0 -1 ];  % exemple si on inverse X et Z

R_cam_3 = [ 0  -1  0;
             1 0  0;
             0  0 1 ];  % exemple si on inverse X et Z

R_cam_0 = R03 * R_cam_3;  % rotation de la caméra dans le global

p_obj_0 = p_cam_0 + R_cam_0 * p_obj_cam;


end

function T = quanser_arm_DH(a,alpha,d,theta)

%% QUANSER_ARM_DH
% v 1.0 - 26th March 2019

% REFERENCE: 
% Chapter 3. Forward and Inverse Kinematics
% Robot Modeling and Control 
% Spong, Hutchinson, Vidyasagar
% 2006

% INPUTS:
% a       :   translation  : along : x_{i}   : from : z_{i-1} : to : z_{i}
% alpha   :      rotation  : about : x_{i}   : from : z_{i-1} : to : z_{i}
% d       :   translation  : along : z_{i-1} : from : x_{i-1} : to : x_{i}
% theta   :      rotation  : about : z_{i-1} : from : x_{i-1} : to : x_{i}
% NOTE: Standard DH Parameters

% OUTPUTS:
% T       : transformation                   : from :     {i} : to : {i-1}

%%
% Rotation Transformation about z axis by theta
T_R_z = [cos(theta) -sin(theta) 0 0;
         sin(theta)  cos(theta) 0 0;
                  0           0 1 0;
                  0           0 0 1];
     
% Translation Transformation along z axis by d
T_T_z = [1 0 0 0;
         0 1 0 0;
         0 0 1 d;
         0 0 0 1];

% Translation Transformation along x axis by a
T_T_x = [1 0 0 a;
         0 1 0 0;
         0 0 1 0;
         0 0 0 1];

% Rotation Transformation about x axis by alpha
T_R_x = [1          0           0 0;
         0 cos(alpha) -sin(alpha) 0;
         0 sin(alpha)  cos(alpha) 0;
         0          0           0 1];

% For a transformation FROM frame {i} TO frame {i-1}: A
T = T_R_z*T_T_z*T_T_x*T_R_x;

end

== matlab function connecttoUDP_Ask_For_Ball/forward kinematics5 ==
  data: xyz input; xyz_mean output
function xyz_mean = mean_xyz_1s(xyz)
% xyz : [3x1] ou [1x3]
% xyz_mean : [3x1] moyenne sur 1 seconde

    %#codegen

    % PARAMÈTRES
    N = 1;   % nombre d'échantillons pour 1 seconde (Ts = 0.01s)

    % PERSISTANTS À TAILLE FIXE
    persistent buffer index count

    if isempty(buffer)
        buffer = zeros(3, N);
        index  = 1;
        count  = 0;
    end

    % Forcer vecteur colonne
    xyz = xyz(:);

    % Stockage circulaire
    buffer(:, index) = xyz;

    index = index + 1;
    if index > N
        index = 1;
    end

    if count < N
        count = count + 1;
    end

    % Moyenne
    xyz_mean = sum(buffer(:,1:count), 2) / count;

end

== matlab function connecttoUDP_Ask_For_Ball/inverse kinematics1 ==
  data: p input; gamma input; phi_optimal output; phi_prev input
function phi_optimal = qarmInverseKinematics(p, gamma, phi_prev)
%% QARM Inverse Kinematics (NaN-safe, limite saturée)
% Si la position exacte n'est pas atteignable, renvoie la configuration
% la plus proche atteignable.
% INPUTS:
%   p        : position [x;y;z] en m
%   gamma    : rotation poignet (rad)
%   phi_prev : configuration précédente [4x1] en rad
% OUTPUT:
%   phi_optimal : configuration atteignable [4x1] rad

%% Paramètres du manipulateur
L1 = 0.1400; L2 = 0.3500; L3 = 0.0500; L4 = 0.2500; L5 = 0.1500;
beta = atan(L3/L2);

lambda1 = L1;
lambda2 = sqrt(L2^2 + L3^2);
lambda3 = L4 + L5;

%% Initialisation
theta = zeros(4,4);
phi   = zeros(4,4);

%% --- Calcul theta2 / theta3 ---
A = lambda2; C = -lambda3; H = lambda1 - p(3);
D1 = -sqrt(p(1)^2 + p(2)^2); 
D2 =  sqrt(p(1)^2 + p(2)^2);

F1 = (D1^2 + H^2 - A^2 - C^2)/(2*A);
F2 = (D2^2 + H^2 - A^2 - C^2)/(2*A);

% Si racine négative, on met la valeur maximale atteignable
if C^2 - F1^2 < 0
    warning('Position non atteignable pour solution 1/2 : saturation');
    theta(3,1) = sign(C)*pi/2;  % valeur maximale atteignable
    theta(3,2) = sign(C)*pi/2;
else
    theta(3,1) = 2*atan2( C + sqrt(C^2 - F1^2), F1 );
    theta(3,2) = 2*atan2( C - sqrt(C^2 - F1^2), F1 );
end

if C^2 - F2^2 < 0
    warning('Position non atteignable pour solution 3/4 : saturation');
    theta(3,3) = sign(C)*pi/2;
    theta(3,4) = sign(C)*pi/2;
else
    theta(3,3) = 2*atan2( C + sqrt(C^2 - F2^2), F2 );
    theta(3,4) = 2*atan2( C - sqrt(C^2 - F2^2), F2 );
end

%% --- Calcul theta2 ---
for i = 1:4
    D = D1; if i>2, D=D2; end
    M = A + C*sin(theta(3,i));
    N = -C*cos(theta(3,i));
    if abs(M)<1e-6, M=sign(M)*1e-6; end
    cos_term = (D*M + H*N)/(M^2 + N^2);
    sin_term = (H - N*cos_term)/M;
    theta(2,i) = atan2(sin_term, cos_term);
end

%% --- Calcul theta1 ---
for i = 1:4
    denom = lambda2*cos(theta(2,i)) - lambda3*sin(theta(2,i)+theta(3,i));
    if abs(denom)<1e-6, denom=sign(denom)*1e-6; end
    theta(1,i) = atan2(p(2)/denom, p(1)/denom);
end

%% --- Remap vers angles QARM ---
phi(1,:) = theta(1,:);
phi(2,:) = theta(2,:) - beta + pi/2;
phi(3,:) = theta(3,:) + beta;
phi(4,:) = gamma;

phi = mod(phi+pi, 2*pi) - pi; % normalisation [-pi,pi]

%% --- Saturation des limites ---
for i=1:4
    phi(:,i) = saturate_joint_limits(phi(:,i));
end

%% --- Choix solution la plus proche de phi_prev ---
phi_optimal = phi(:,1);
best_norm = norm(phi(:,1)-phi_prev);
for i=2:4
    current_norm = norm(phi(:,i)-phi_prev);
    if current_norm < best_norm
        phi_optimal = phi(:,i);
        best_norm = current_norm;
    end
end

end

%% --- Fonction de saturation ---
function phi_sat = saturate_joint_limits(phi)
limits = [
    -170  170;
    -80    80;
    -95    75;
    -160  160
]*pi/180;

phi_sat = phi;
for i=1:4
    if phi(i)<limits(i,1), phi_sat(i)=limits(i,1); end
    if phi(i)>limits(i,2), phi_sat(i)=limits(i,2); end
end
end

== matlab function connecttoUDP_Ask_For_Ball/inverse kinematics2 ==
  data: p input; gamma input; phi_optimal output; phi_prev input
function phi_optimal = qarmInverseKinematics(p, gamma, phi_prev)

%% QUANSER_ARM_IPK
% v 4.0 - 4th June 2020

% REFERENCE: 
% Chapter 4. Inverse Kinematics
% Robot Dynamics and Control 
% Spong, Vidyasagar
% 1989

% INPUTS:
% p        : end-effector position vector expressed in base frame {0}
% gamma    : wrist rotation angle gamma

% OUTPUTS:
% phi_optimal : Best solution depending on phi_prev
% phi         : All four Inverse Kinematics solutions as a 4x4 matrix. 
%               Each col is a solution.

%% Manipulator parameters:
L1 = 0.1400;
L2 = 0.3500;
L3 = 0.0500;
L4 = 0.2500;
L5 = 0.1500;
beta = atan(L3/L2);

%% Alternate parameters
lambda1 = L1;
lambda2 = sqrt(L2^2 + L3^2);
lambda3 = L4 + L5;

%% Initialization
theta   = zeros(4, 4);
phi = zeros(4, 4);

%% Joint angle 2 and 3: 
% Equations:
    % lambda2 cos(theta2) + (-lambda3) sin(theta2 + theta3) = sqrt(x^2 + y^2)
    %   A     cos( 2    ) +     C      sin(   2   +    3  ) =    D
    
    % lambda2 sin(theta2) - (-lambda3) cos(theta2 + theta3) = lambda1 - z
    %   A     sin( 2    ) -     C      cos(   2   +    3  ) =    H

% Solution:
    A = lambda2;
    C = -lambda3;
    H =  lambda1 - p(3);
    D1 = -sqrt(p(1)^2 + p(2)^2);
    D2 = sqrt(p(1)^2 + p(2)^2);
    F = (D1^2 + H^2 - A^2 - C^2)/(2*A);

    theta(3,1) = 2*atan2( C + sqrt(C^2 - F^2) , F );
	theta(3,2) = 2*atan2( C - sqrt(C^2 - F^2) , F );
    theta(3,3) = 2*atan2( C + sqrt(C^2 - F^2) , F );
	theta(3,4) = 2*atan2( C - sqrt(C^2 - F^2) , F );

    M = A + C*sin(theta(3,1));
    N = -C*cos(theta(3,1));
    cos_term = (D1*M + H*N)/(M^2 + N^2);
    sin_term = (H - N*cos_term)/(M);
    theta(2,1) = atan2(sin_term, cos_term);

    M = A + C*sin(theta(3,2));
    N = -C*cos(theta(3,2));
    cos_term = (D1*M + H*N)/(M^2 + N^2);
    sin_term = (H - N*cos_term)/(M);
    theta(2,2) = atan2(sin_term, cos_term);

    M = A + C*sin(theta(3,3));
    N = -C*cos(theta(3,3));
    cos_term = (D2*M + H*N)/(M^2 + N^2);
    sin_term = (H - N*cos_term)/(M);
    theta(2,3) = atan2(sin_term, cos_term);

    M = A + C*sin(theta(3,4));
    N = -C*cos(theta(3,4));
    cos_term = (D2*M + H*N)/(M^2 + N^2);
    sin_term = (H - N*cos_term)/(M);
    theta(2,4) = atan2(sin_term, cos_term);


%% Joint angle 1:
% Equation:
    % y / x = tan(theta1);

% Solution
    theta(1,1) = atan2( p(2)/( lambda2 * cos( theta(2,1) ) - lambda3 * sin( theta(2,1) + theta(3,1) ) ) , p(1)/(  lambda2 * cos( theta(2,1) ) - lambda3 * sin( theta(2,1) + theta(3,1) )  ) );
    theta(1,2) = atan2( p(2)/( lambda2 * cos( theta(2,2) ) - lambda3 * sin( theta(2,2) + theta(3,2) ) ) , p(1)/(  lambda2 * cos( theta(2,2) ) - lambda3 * sin( theta(2,2) + theta(3,2) )  ) );
    theta(1,3) = atan2( p(2)/( lambda2 * cos( theta(2,3) ) - lambda3 * sin( theta(2,3) + theta(3,3) ) ) , p(1)/(  lambda2 * cos( theta(2,3) ) - lambda3 * sin( theta(2,3) + theta(3,3) )  ) );
    theta(1,4) = atan2( p(2)/( lambda2 * cos( theta(2,4) ) - lambda3 * sin( theta(2,4) + theta(3,4) ) ) , p(1)/(  lambda2 * cos( theta(2,4) ) - lambda3 * sin( theta(2,4) + theta(3,4) )  ) );
    
%% Remap theta back to phi
% phi(1) = theta(1);
% phi(2) = theta(2) - beta + pi/2;
% phi(3) = theta(3) + beta;
% phi(4) = theta(4);

phi(1,:) = theta(1,:);
phi(2,:) = theta(2,:) - beta + pi/2;
phi(3,:) = theta(3,:) + beta;
phi(4,:) = gamma;

phi = mod(phi + pi, 2*pi) - pi;

phi_optimal = phi(:,1);
if (norm(phi_optimal - phi_prev) > norm(phi(:,2) - phi_prev)) || (check_joint_limits(phi_optimal))
    phi_optimal = phi(:,2);
end
if (norm(phi_optimal - phi_prev) > norm(phi(:,3) - phi_prev)) || (check_joint_limits(phi_optimal))
    phi_optimal = phi(:,3);
end
if (norm(phi_optimal - phi_prev) > norm(phi(:,4) - phi_prev)) || (check_joint_limits(phi_optimal))
    phi_optimal = phi(:,4);
end
if (check_joint_limits(phi_optimal))
    phi_optimal = [0;0;0;0];
end

end

function flag = check_joint_limits(phi)
    flag = 0;
    if phi(1) > 170*pi/180 || phi(1) < -170*pi/180 ...
        || phi(2) > 85*pi/180 || phi(2) < -85*pi/180 ... 
        || phi(3) > 75*pi/180 || phi(3) < -95*pi/180 ...
        || phi(4) > 160*pi/180 || phi(4) < -160*pi/180
    flag = 1;
    end
end
